simulink model "vipabandonedobj_bayer_hwcs_replaced_inputs_outputs"  (Simulink 10.0)
settings: Solver=ode45  StartTime=0.0  StopTime=500000  RelTol=1e-3  EnableMultiTasking=on
StartFcn:
  | tic
StopFcn:
  | toc
undefined symbols (not defined in the file): A8C0F68A, BBA0, Device, E2E8303F83B4, NPF_
libraries: xbsIndex_r4 x3, dspbuff3 x2, S3ADSP_SK_PPEth_RuntimeCosim x1
settings Model: Creator=thill  LastModifiedBy=bhisma
settings DataIOCC: LimitDataPoints=on  SignalLoggingSaveFormat=ModelDataLogs
settings OptimizationCC: ExpressionDepthLimit=2147483647  InitFltsAndDblsToZero=on
settings DebuggingCC: SaveWithParameterizedLinksMsg=none  SolverPrmCheckMsg=warning  FcnCallInpInsideContextMsg=warning  StateNameClashWarn=warning
settings SFSimCC: SimUseLocalCustomCode=on  CustomCodeUndefinedFunction=FilterOut
settings RTWCC: RTWUseLocalCustomCode=on
settings GRTTargetCC: TargetFcnLib=ansi_tfl_tmw.mat

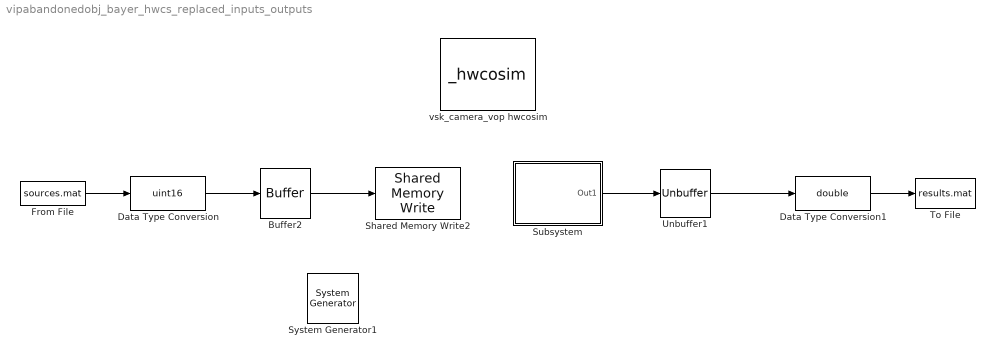
== system vipabandonedobj_bayer_hwcs_replaced_inputs_outputs ==
  " System Generator1" : xbsIndex_r4/ System Generator  Tag=genX  SystemSampleTime=-1  xilinxfamily=virtex4  part=xc4vsx35  speed=-10  package=ff668  synthesis_tool=XST  directory=./netlist  testbench=off  simulink_period=2880  sysclk_period=10  incr_netlist=off  trim_vbits=Everywhere in SubSystem  dbl_ovrd=According to Block Masks  core_generation=According to Block Masks  run_coregen=off  deprecated_control=off  eval_field=0  block_type=sysgen
      settings: block_version=9.2.01
  Buffer2 : dspbuff3/Buffer  N=2880  V=0  ic=0
      settings: SourceProductName=DSP System Toolbox  SourceProductBaseCode=DS
  Data Type Conversion : DataTypeConversion  OutDataTypeStr=uint16
  Data Type Conversion1 : DataTypeConversion  OutDataTypeStr=double
  From File : FromFile  FileName=sources.mat  SampleTime=1
  Shared Memory Write2 : xbsIndex_r4/Shared Memory Write  Priority=2  shmem_name='data_in'  shmem_type=FIFO  skip_check=on  shmem_word=16  shmem_depth=4095  block_type=toshmem
      settings: AttributesFormatString=<< %<shmem_name> >>  infoedit=Writes scalar, vector, matrix, or frame data into a shared memory.  block_version=VER_STRING_GOES_HERE
  Subsystem : Subsystem
  To File : ToFile  Filename=results.mat
  Unbuffer1 : dspbuff3/Unbuffer  ic=0
      settings: SourceProductName=DSP System Toolbox  SourceProductBaseCode=DS
  vsk_camera_vop hwcosim : S3ADSP_SK_PPEth_RuntimeCosim/_hwcosim  clkSrc=Free Running  hasCombinationalPath=on  bitfileName=C:\hill\WWM\seminars\mathworks_vsk\seminar_designs\hw_cosim\netlist\sp3dsp1800\vsk_camera_vop_cw.bit  ethernetInterface=Please select an Ethernet interface  fpgaEthernetAddr=00:0a:35:11:22:33  cable=Xilinx Parallel Cable IV  speed=5 MHz  configTimeout=3000  treeview=|  design_xtable=|  cosim_xtable={'ethernetCosim'=>{'bscanPos'=>1,'maxFrameSize'=>2040,'target'=>'S3ADSP_SK','type'=>'ppethernet'}}  ethernetInterfaceID=\Device\NPF_{A8C0F68A-51F8-4EB4-BBA0-E2E8303F83B4}  useWaitBox=1  prgClkFreq=50  bscanPos=1  Scheme=Cosim  memxtable={'treeview'=>[{'icon'=>'fifo','label'=>'&lt;&lt;&apos;data_in&apos;&gt;&gt;','param'=>['Depth: 4095','Number of Bits: 16','Type: From FIFO'],'state'=>0.00000000000000000},{'icon'=>'fifo','label'=>'&lt;&lt;&apos;data_out&apos;&gt;&gt;','param'=>['Depth: 4095','Number of Bits: 32','Type: To FIFO'],'state'=>0.00000000000000000}]}  hasProc=0  block_type=ppethernet_cosim
      treeview=|
      | <html><head><meta name="qrichtext" content="1" /><style type="text/css">
      | p, li { white-space: pre-wrap; }
      | </style></head><body style=" font-family:'MS Shell Dlg 2'; font-size:8.25pt; font-weight:400; font-style:normal;" bgcolor="#ffffff">
      | <p style=" margin-top:0px; margin-bottom:0px; margin-left:0px; margin-right:0px; -qt-block-indent:0; text-indent:0px; font-size:8pt;"><img src="C:\Xilinx\dsptools\9.2.01.1028\sysgen\data\images\fifoplus.gif" />&lt;&lt;'data_in'&gt;&gt;<br /></p>
      | <p style=" margin-top:0px; margin-bottom:0px; margin-left:0px; margin-right:0px; -qt-block-indent:0; text-indent:0px; font-size:8pt;"><img src="C:\Xilinx\dsptools\9.2.01.1028\sysgen\data\images\fifoplus.gif" />&lt;&lt;'data_out'&gt;&gt;<br /></p></body></html>
      design_xtable=|
      | {
      |   'clkWrapper' => 'vsk_camera_vop_cw',
      |   'clocksGcd' => 1,
      |   'device' => 'xc3sd1800a-4fg676',
      |   'ports' => {},
      |   'shared_memories' => {
      |     'data_in' => {
      |       'bank' => 0,
      |       'block_config' => 'sysgen_blockset:fromfifo_config',
      |       'data_addr' => 0,
      |       'depth' => 4095,
      |       'full_empty_index' => 0,
      |       'percent_full_index' => 1,
      |       'width' => 16,
      |     },
      |     'data_out' => {
      |       'bank' => 0,
      |       'block_config' => 'sysgen_blockset:tofifo_config',
      |       'data_addr' => 2,
      |       'depth' => 4095,
      |       'full_empty_index' => 4,
      |       'percent_full_index' => 5,
      |       'width' => 32,
      |     },
      |   },
      | }
      settings: block_version=9.2.01
  wires:
  Buffer2/1 -> Shared Memory Write2/1
  Unbuffer1/1 -> Data Type Conversion1/1
  Subsystem/1(Out1) -> Unbuffer1/1
  From File/1 -> Data Type Conversion/1
  Data Type Conversion/1 -> Buffer2/1
  Data Type Conversion1/1 -> To File/1

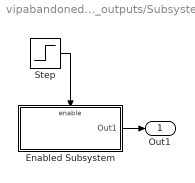
== system vipabandonedobj_bayer_hwcs_replaced_inputs_outputs/Subsystem ==
  Enabled Subsystem : Subsystem  TreatAsAtomicUnit=on
  Step : Step  SampleTime=0
  Out1 : Outport
  wires:
  Step/1 -> Enabled Subsystem/Enable
  Enabled Subsystem/1(Out1) -> Out1/1

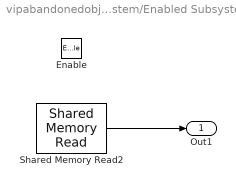
== system vipabandonedobj_bayer_hwcs_replaced_inputs_outputs/Subsystem/Enabled Subsystem ==
  Enable : EnablePort
  Shared Memory Read2 : xbsIndex_r4/Shared Memory Read  Priority=20  shmem_name='data_out'  shmem_type=FIFO  sample_time=2880  dataType=uint32  outDims=[2880 1]  isFrame=on  shmem_word=32  shmem_depth=4095  block_type=fromshmem
      settings: AttributesFormatString=<< %<shmem_name> >>  infoedit=Reads sequentially from a shared memory block.  block_version=VER_STRING_GOES_HERE
  Out1 : Outport
  wires:
  Shared Memory Read2/1 -> Out1/1
